simulink model "l18_ex1"  (R2018b)
settings: Solver=ode45  StartTime=0.0  StopTime=7  MaxStep=1e-4  RelTol=1e-4  AbsTol=1e-4  EnableMultiTasking=on
values from neighbouring files (symbols this model uses):
  Kd = 2    [l16.m]    (also in l18.m = 0.031)
  Ki = Ki_list(k)    [l15.m]    (also in l18.m = 5.65)
  Kp = Kp_list(k)    [l15.m]    (also in l16.m = 8; l18.m = 0.372)
settings Model: Creator=Joe  LastModifiedBy=joema
settings SolverCC: AutoScaleAbsTol=off
settings DataIOCC: LimitDataPoints=on  SaveFormat=Array
settings OptimizationCC: LifeSpan=inf
settings DebuggingCC: UnderspecifiedInitializationDetection=Classic  MergeDetectMultiDrivingBlocksExec=none  LibraryContextMissingDiagnostic=none  SFUnexpectedBacktrackingDiag=warning  SFNoUnconditionalDefaultTransitionDiag=warning  SFExecutionAtInitializationDiag=none
settings HardwareCC: ProdBitPerPointer=32  ProdBitPerSizeT=32  ProdBitPerPtrDiffT=32  ProdLargestAtomicFloat=None  ProdIntDivRoundTo=Undefined  ProdEndianess=Unspecified  ProdWordSize=32  ProdHWDeviceType=32-bit Generic
settings ModelReferenceCC: PropagateSignalLabelsOutOfModel=off
settings SFSimCC: SimUseLocalCustomCode=off
settings RTWCC: RTWUseLocalCustomCode=off
settings CodeAppCC: StateflowObjectComments=on
settings GRTTargetCC: TargetLangStandard=C89/C90 (ANSI)  GeneratePreprocessorConditionals=Disable all
settings ConfigComp: CovMetricSettings=dw  CovHtmlReporting=on  CovSaveCumulativeToWorkspaceVar=on  CovSaveSingleToWorkspaceVar=on  CovExternalEMLEnable=off  CovSFcnEnable=off

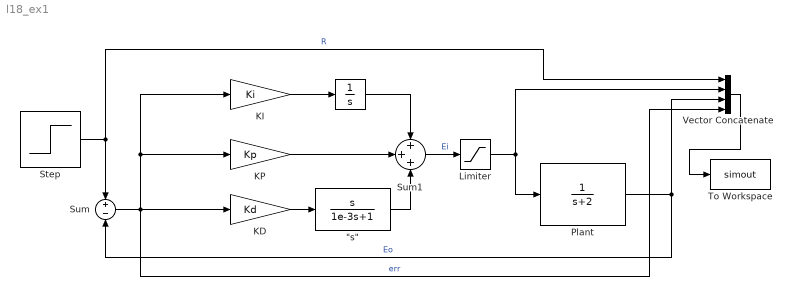
== system l18_ex1 ==
  " " : Integrator
  "\"s\"" : TransferFcn  Numerator=[1 0]  Denominator=[1e-3 1]
  KD : Gain  Gain=Kd
  KI : Gain  Gain=Ki
  KP : Gain  Gain=Kp
  Limiter : Saturate  UpperLimit=20  LowerLimit=-20
  Plant : TransferFcn  Denominator=[1 2]
  Step : Step  Time=0  After=5  SampleTime=0
  Sum : Sum  Inputs=+-
  Sum1 : Sum  Inputs=+++
  To Workspace : ToWorkspace  VariableName=simout  SaveFormat=Timeseries  SampleTime=-1
  Vector Concatenate : Concatenate  NumInputs=4
  wires:
  Step/1 -> Sum/1, Vector Concatenate/1  "R"
  Plant/1 -> Sum/2, Vector Concatenate/3  "Eo"
  Vector Concatenate/1 -> To Workspace/1
  Sum/1 -> Vector Concatenate/4, KP/1, KI/1, KD/1  "err"
  KP/1 -> Sum1/2
  KI/1 -> " "/1
  " "/1 -> Sum1/1
  KD/1 -> "\"s\""/1
  "\"s\""/1 -> Sum1/3
  Sum1/1 -> Limiter/1  "Ei"
  Limiter/1 -> Vector Concatenate/2, Plant/1
